simulink model "SF015A_WhlImbRejctn"  (R2013b)
settings: Solver=FixedStepDiscrete  SolverMode=SingleTasking  StartTime=0.0  StopTime=1  FixedStep=0.002  RelTol=1e-3
undefined symbols (not defined in the file): ACTIVBANDMAX_ULS_U32, ADAPVFILMAX_ULS_F32, ADJOUTPMAX_ULS_F32, ARCHGLBPRM_180OVERPI_ULS_F32, ARCHGLBPRM_2MILLISEC_SEC_F32, ARCHGLBPRM_2PI_ULS_F32, ARCHGLBPRM_FLOATZEROTHD_ULS_F32, ARCHGLBPRM_PI_ULS_F32, ARCHGLBPRM_PIOVER180_ULS_F32, ARCHGLBPRM_PIOVER2_ULS_F32, CALMINSPERCOUNT_ULS_F32, Cntr, DURATIONDISABLE_CNT_U16, FILTWHLSPDMAX_MOTRADPERSEC_F32, FRQMIN_ULS_F32, MICROSECTOMILLISEC_ULS_F32, MINSTOMILLISEC_ULS_F32, NINETY_ULS_F32, NODEBSTEP_CNT_U16, NROFDLY_CNT_U08, NtcSts1, NvmGetErrSts1, ONEHALF_ULS_F32, ONEHUNDRED_ULS_F32, ONEOVRTHREE_ULS_F32, ONEOVRTWENTY_ULS_F32, ONETHOUSAND_ULS_F32, PEAKMAX_ULS_F32, PEAKMIN_ULS_F32, PHAADJMAX_ULS_F32, PITIMESSAMPLETIME_ULS_F32, SigQlfr1, STOREDMINSPERCOUNT_ULS_F32, Sts, SysSt1, TWO_ULS_F32, TWOOVRTHREE_ULS_F32, UGRFILMAX_ULS_F32, WhlImbRejctnAdpvFac, WhlImbRejctnAutScaEna, WhlImbRejctnAutScaTar, WhlImbRejctnCurrMgnSlewPerLoop, WhlImbRejctnDcTrendFltRcvryDly, WhlImbRejctnDcTrendFltRcvryNegStep, WhlImbRejctnDcTrendFltRcvryPosStep, WhlImbRejctnDcTrendFltRcvryThd, WhlImbRejctnDcTrendTh2Tq, WhlImbRejctnDcTrendThTq, WhlImbRejctnDcTrendTi2Sec, WhlImbRejctnDcTrendTiSec, WhlImbRejctnEnaSlewPerLoop, WhlImbRejctnFctEna, WhlImbRejctnFltNtc, WhlImbRejctnFrqDiagcAmpThd, WhlImbRejctnFrqDiagcEna, WhlImbRejctnFrqDiagcFltRcvryDly, WhlImbRejctnFrqDiagcFltRcvryNegStep, WhlImbRejctnFrqDiagcFltRcvryPosStep, WhlImbRejctnFrqDiagcFltRcvryThd, WhlImbRejctnFrqDiagcThd ... (+30)
libraries: FixdToFloat x32, simulink x26, NxtrLim x25, Fil x20, NxtrAbslt x9, NxtrMath x7, NxtrMax x6, NxtrMin x4, NxtrNvM x2, FloatToFixd x2, LnrIntrpn x2, NxtrSign x1
(part 2 of 14)

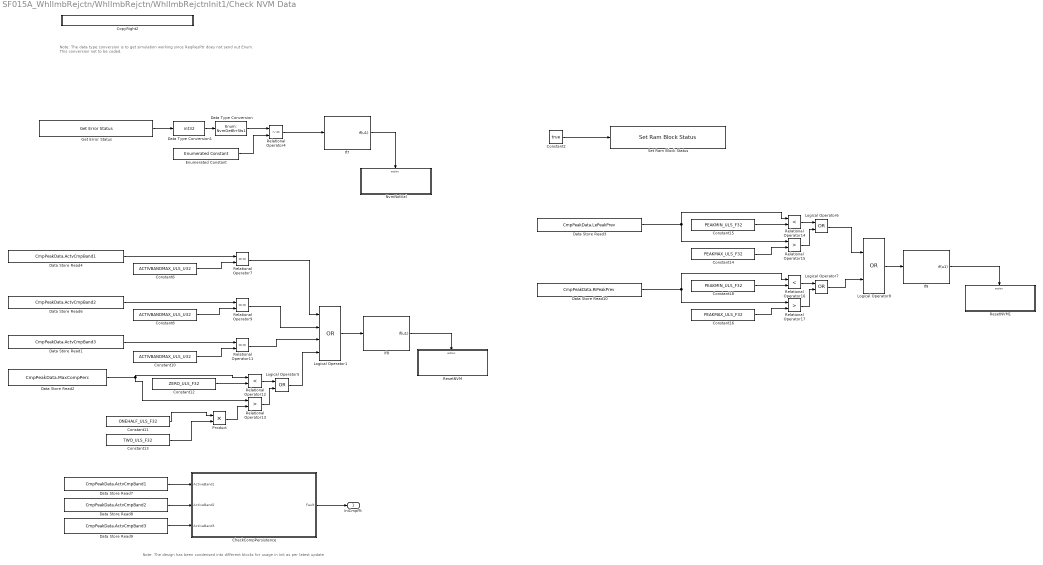
== system SF015A_WhlImbRejctn/WhlImbRejctn/WhlImbRejctnInit1/Check NVM Data ==
  note: Note: The data type conversion is to get simulation working since ReqResPtr does not send out Enum. This
      | conversion not to be coded.
  note: Note: The design has been condensed into different blocks for usage in Init as per latest update
  CheckCompPersistence : Subsystem
  Constant10 : Constant  RequirementInfo={} %GIDa_dac22d33_84e0_4d43_9baa_6580695156ec  Value=ACTIVBANDMAX_ULS_U32
  Constant11 : Constant  RequirementInfo={} %GIDa_b70b5de3_e4e7_4656_8a10_81d881ba1c41  Value=ONEHALF_ULS_F32
  Constant12 : Constant  RequirementInfo={} %GIDa_d9980660_ddd4_4231_a48f_0f3c433b1d8f  Value=ZERO_ULS_F32
  Constant13 : Constant  RequirementInfo={} %GIDa_8a202516_8579_4314_b780_b551ef6a9ea7  Value=TWO_ULS_F32
  Constant14 : Constant  RequirementInfo={} %GIDa_73aa9993_742b_457a_81a0_f953eb76670e  Value=PEAKMAX_ULS_F32
  Constant15 : Constant  RequirementInfo={} %GIDa_1412b3b4_8a5a_4483_b46c_39b8aea63137  Value=PEAKMIN_ULS_F32
  Constant16 : Constant  RequirementInfo={} %GIDa_fb2105b3_9180_4cca_ab02_2c62039e61f3  Value=PEAKMAX_ULS_F32
  Constant18 : Constant  RequirementInfo={} %GIDa_e66c83e2_3c4a_4c53_aaa1_18a5c79d3e74  Value=PEAKMIN_ULS_F32
  Constant2 : Constant  Value=true  OutDataTypeStr=boolean
      settings: AttributesFormatString=%<OutDataTypeStr>
  Constant6 : Constant  RequirementInfo={} %GIDa_8360f5ba_58c9_48ae_bbc1_d6eb240405df  Value=ACTIVBANDMAX_ULS_U32
  Constant8 : Constant  RequirementInfo={} %GIDa_5c7deeb0_1ebc_45b4_93cb_ec8df33bc324  Value=ACTIVBANDMAX_ULS_U32
  CopyRight2 : Subsystem  Description=|  mask(Copyright Information){none=on}
      | Copyright info block.                                               
      |                                                                     
      | Place copyright information at the top of every subsystem in design.
      mask prompts: none "No parameters"
      mask help: Place copyright information at the top of every subsystem in design.
      mask Display:
      | NxtrConf = 'Nexteer Confidential';
      | 
      | sys = bdroot; %handle for the current model ("system")
      | first = get_param(sys,'Created');
      | first = first(end-3:end);  %year is last four digits
      | 
      | last = get_param(sys,'LastModifiedDate');
      | if isempty(last)
      |     last = datestr(now,'yyyy');
      | else
      |     last = last(end-3:end);
      | end
      | 
      | if strcmp(first,last)
      |     fprintf('%s -- Copyright %s Nexteer',NxtrConf,first)
      | else
      |     fprintf('%s -- %s%s- %s Nexteer',NxtrConf,char(169),first,last)
      | end
  Data Store Read1 : DataStoreRead  RequirementInfo={} %GIDa_9fdfabdd_f7fe_4007_8b29_7d33a37c1ea7  DataStoreName=CmpPeakData  DataStoreElements=CmpPeakData.ActvCmpBand3
  Data Store Read10 : DataStoreRead  RequirementInfo={} %GIDa_8b90afc5_6e2e_402d_8a16_4fba91ced75f  DataStoreName=CmpPeakData  DataStoreElements=CmpPeakData.RiPeakPrev
  Data Store Read2 : DataStoreRead  RequirementInfo={} %GIDa_c9bc2b23_4b2d_4415_bc50_be739cb942b2  DataStoreName=CmpPeakData  DataStoreElements=CmpPeakData.MaxCompPerc
  Data Store Read3 : DataStoreRead  RequirementInfo={} %GIDa_b09638af_4375_4cc5_b3f9_eff43fa8b240  DataStoreName=CmpPeakData  DataStoreElements=CmpPeakData.LePeakPrev
  Data Store Read4 : DataStoreRead  RequirementInfo={} %GIDa_a896886f_cd25_4b88_9045_5429e28523e8  DataStoreName=CmpPeakData  DataStoreElements=CmpPeakData.ActvCmpBand1
  Data Store Read6 : DataStoreRead  RequirementInfo={} %GIDa_0bac01f8_9053_4f69_a3f3_2d14815d55fa  DataStoreName=CmpPeakData  DataStoreElements=CmpPeakData.ActvCmpBand2
  Data Store Read7 : DataStoreRead  Priority=3  DataStoreName=CmpPeakData  DataStoreElements=CmpPeakData.ActvCmpBand1
      settings: AttributesFormatString=Priority=%<Priority>
  Data Store Read8 : DataStoreRead  Priority=3  DataStoreName=CmpPeakData  DataStoreElements=CmpPeakData.ActvCmpBand2
      settings: AttributesFormatString=Priority=%<Priority>
  Data Store Read9 : DataStoreRead  Priority=3  DataStoreName=CmpPeakData  DataStoreElements=CmpPeakData.ActvCmpBand3
      settings: AttributesFormatString=Priority=%<Priority>
  Data Type Conversion : DataTypeConversion  RequirementInfo={} %GIDa_40af021a_ef54_4ec7_b6de_237be91b60fa  OutDataTypeStr=Enum: NvmGetErrSts1
  Data Type Conversion1 : DataTypeConversion  RequirementInfo={} %GIDa_97cfbfab_5bcd_4235_a187_9f25ba5a5ff5  OutDataTypeStr=int32
  Enumerated Constant : simulink/Sources/Enumerated Constant  RequirementInfo={} %GIDa_d56addf7_f0d4_4bf6_af4c_9a6eaaf5d064  OutDataTypeStr=Enum: NvmGetErrSts1  Value=NvmGetErrSts1.REQUEST_OK  SampleTime=inf
  Get Error Status : NxtrNvM/Get Error Status  RequirementInfo={} %GIDa_553b790d_fe60_40ec_8b91_d9fbb8c02471  FuncName=Get Error Status  NvMBlockName=CmpPeakData  VoidFuncRtn=on  ReqResPtr_DSN=NvMGES_ReqResPtr1  Return_DSN=NvMGES_Return
      settings: AttributesFormatString=%<FuncName>
  If7 : If  RequirementInfo={} %GIDa_907c88cf_d2cc_420d_8539_4883f54d5bfb  Priority=0  IfExpression=u1  ShowElse=off
  If8 : If  RequirementInfo={} %GIDa_f83260c7_70fe_47e6_bcfd_8d40190318cc  Priority=0  IfExpression=u1  ShowElse=off
  If9 : If  RequirementInfo={} %GIDa_2d76ece9_77c8_4d3b_9932_2561659afd1c  Priority=0  IfExpression=u1  ShowElse=off
  Logical Operator1 : Logic  RequirementInfo={} %GIDa_6b27fa6d_5a8c_4b6e_9ec1_9ce35c4a7e3a  Operator=OR  Inputs=4  AllPortsSameDT=off  OutDataTypeStr=boolean
  Logical Operator5 : Logic  RequirementInfo={} %GIDa_ff21cde4_e337_434b_869a_bfcb48407868  Operator=OR  AllPortsSameDT=off  OutDataTypeStr=boolean
  Logical Operator6 : Logic  RequirementInfo={} %GIDa_22490e7d_9c19_4dde_99cc_08f0ef37cc37  Operator=OR  AllPortsSameDT=off  OutDataTypeStr=boolean
  Logical Operator7 : Logic  RequirementInfo={} %GIDa_0952c7bd_6ac0_4128_a8d2_c4d9c59f71ec  Operator=OR  AllPortsSameDT=off  OutDataTypeStr=boolean
  Logical Operator8 : Logic  RequirementInfo={} %GIDa_f87f89e5_1919_41e6_b4c5_1617d795e711  Operator=OR  AllPortsSameDT=off  OutDataTypeStr=boolean
  NvmNotVal : Subsystem  RequirementInfo={} %GIDa_f6393af9_0f72_404f_ae39_57d92493339f  TreatAsAtomicUnit=on
  Product : Product
  Relational Operator11 : RelationalOperator  RequirementInfo={} %GIDa_9bbcc360_5740_4f1b_a35a_ba783374856a  Operator===  OutDataTypeStr=boolean
  Relational Operator12 : RelationalOperator  RequirementInfo={} %GIDa_a76e833d_5218_4e43_8d52_6f49a79e2f35  Operator=<  OutDataTypeStr=boolean
  Relational Operator13 : RelationalOperator  RequirementInfo={} %GIDa_4a8bae17_bbe3_48ac_9e0a_4fe9b537a9c6  Operator=>  OutDataTypeStr=boolean
  Relational Operator14 : RelationalOperator  RequirementInfo={} %GIDa_654c4bba_0100_4331_8452_58d1590c8b97  Operator=<  OutDataTypeStr=boolean
  Relational Operator15 : RelationalOperator  RequirementInfo={} %GIDa_e495d182_ff98_497d_82f4_fbf92eddef9e  Operator=>  OutDataTypeStr=boolean
  Relational Operator16 : RelationalOperator  RequirementInfo={} %GIDa_956274a6_c5b5_492b_bac4_f5c4aafd6507  Operator=<  OutDataTypeStr=boolean
  Relational Operator17 : RelationalOperator  RequirementInfo={} %GIDa_3a72db96_6452_4e24_94d0_249eb710d610  Operator=>  OutDataTypeStr=boolean
  Relational Operator4 : RelationalOperator  RequirementInfo={} %GIDa_240ffe86_9b38_40e3_a7e4_d3f8c5427260  Operator=~=  OutDataTypeStr=boolean
  Relational Operator7 : RelationalOperator  RequirementInfo={} %GIDa_ed9b8f8a_c888_45f6_bfd8_2fd8844e647e  Operator===  OutDataTypeStr=boolean
  Relational Operator9 : RelationalOperator  RequirementInfo={} %GIDa_5b0fe435_eb00_4504_b67e_fcbdb6466ad9  Operator===  OutDataTypeStr=boolean
  ResetNVM : Subsystem  RequirementInfo={} %GIDa_841a7b4b_65c9_4d3a_ad5a_ef4b7fb654a5  TreatAsAtomicUnit=on
  ResetNVM1 : Subsystem  RequirementInfo={} %GIDa_21072be2_221d_447f_a6c4_95766f8093de  TreatAsAtomicUnit=on
  Set Ram Block Status : NxtrNvM/Set Ram Block Status  FuncName=Set Ram Block Status  NvMBlockName=CmpPeakData  VoidFuncRtn=on  BlockChanged_DSN=NvMSRBS_BlockChanged1  Return_DSN=NvMSRBS_Return
  IniCmpFlt : Outport
  wires:
  Data Type Conversion/1 -> Relational Operator4/1
  Enumerated Constant/1 -> Relational Operator4/2
  Data Type Conversion1/1 -> Data Type Conversion/1
  Get Error Status/1 -> Data Type Conversion1/1
  Constant6/1 -> Relational Operator7/2
  Relational Operator7/1 -> Logical Operator1/1
  Constant8/1 -> Relational Operator9/2
  Constant10/1 -> Relational Operator11/2
  Logical Operator1/1 -> If8/1
  Data Store Read2/1 -> Relational Operator12/1, Relational Operator13/1
  Constant11/1 -> Product/1
  Constant12/1 -> Relational Operator12/2
  Relational Operator12/1 -> Logical Operator5/1
  Relational Operator13/1 -> Logical Operator5/2
  Logical Operator5/1 -> Logical Operator1/4
  Product/1 -> Relational Operator13/2
  Constant13/1 -> Product/2
  Data Store Read3/1 -> Relational Operator15/1, Relational Operator14/1
  Constant14/1 -> Relational Operator15/2
  Constant15/1 -> Relational Operator14/2
  Relational Operator14/1 -> Logical Operator6/1
  Relational Operator15/1 -> Logical Operator6/2
  Logical Operator6/1 -> Logical Operator8/1
  Data Store Read10/1 -> Relational Operator16/1, Relational Operator17/1
  Constant16/1 -> Relational Operator17/2
  Constant18/1 -> Relational Operator16/2
  Relational Operator16/1 -> Logical Operator7/1
  Relational Operator17/1 -> Logical Operator7/2
  Logical Operator7/1 -> Logical Operator8/2
  Logical Operator8/1 -> If9/1
  Relational Operator9/1 -> Logical Operator1/2
  Relational Operator11/1 -> Logical Operator1/3
  If7/1 -> NvmNotVal/Action
  If8/1 -> ResetNVM/Action
  If9/1 -> ResetNVM1/Action
  Data Store Read7/1 -> CheckCompPersistence/1(ActiveBand1)
  Data Store Read8/1 -> CheckCompPersistence/2(ActiveBand2)
  Data Store Read9/1 -> CheckCompPersistence/3(ActiveBand3)
  CheckCompPersistence/1(Fault) -> IniCmpFlt/1
  Data Store Read4/1 -> Relational Operator7/1
  Data Store Read6/1 -> Relational Operator9/1
  Data Store Read1/1 -> Relational Operator11/1
  Constant2/1 -> Set Ram Block Status/1
  Relational Operator4/1 -> If7/1

== system SF015A_WhlImbRejctn/WhlImbRejctn/WhlImbRejctnInit1/CopyRight2 ==

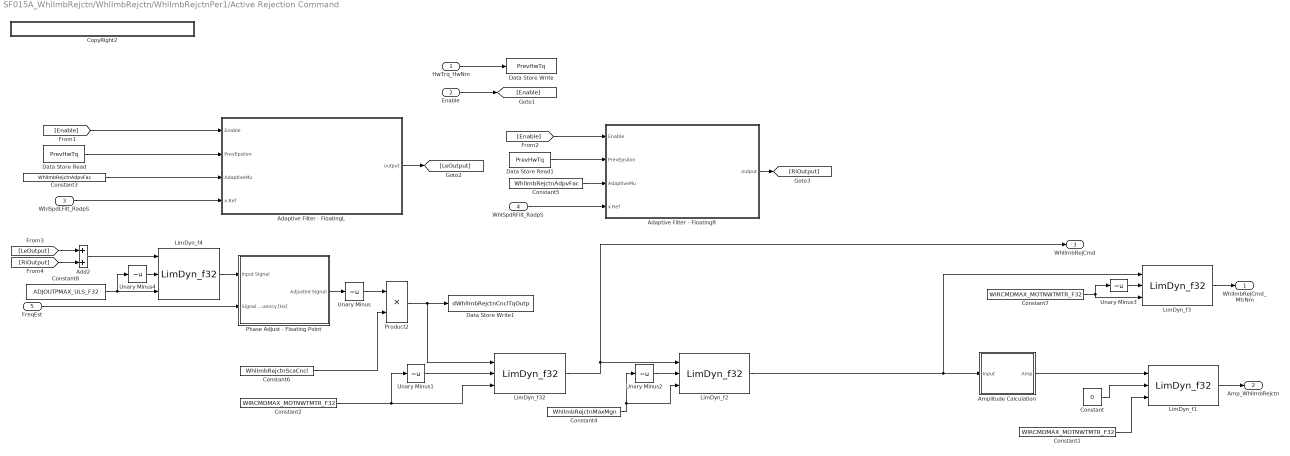
== system SF015A_WhlImbRejctn/WhlImbRejctn/WhlImbRejctnPer1/Active Rejection Command  ==
  HwTrq_HwNm : Inport
  Enable : Inport  Port=2
  WhlSpdLFilt_RadpS : Inport  Port=3
  WhlSpdRFilt_RadpS : Inport  Port=4
  FreqEst : Inport  Port=5
  Adaptive Filter - FloatingL : Subsystem
  Adaptive Filter - FloatingR : Subsystem
  Add2 : Sum
  Amplitude Calculation : Subsystem
  Constant : Constant  Value=0  OutDataTypeStr=single
  Constant1 : Constant  Value=WIRCMDMAX_MOTNWTMTR_F32
  Constant2 : Constant  Value=WIRCMDMAX_MOTNWTMTR_F32
  Constant3 : Constant  Value=WhlImbRejctnAdpvFac
  Constant4 : Constant  Value=WhlImbRejctnMaxMgn
  Constant5 : Constant  Value=WhlImbRejctnAdpvFac
  Constant6 : Constant  Value=WhlImbRejctnScaCncl
  Constant7 : Constant  Value=WIRCMDMAX_MOTNWTMTR_F32
  Constant8 : Constant  Value=ADJOUTPMAX_ULS_F32
  CopyRight2 : Subsystem  Description=|  mask(Copyright Information){none=on}
      | Copyright info block.                                               
      |                                                                     
      | Place copyright information at the top of every subsystem in design.
      mask prompts: none "No parameters"
      mask help: Place copyright information at the top of every subsystem in design.
      mask Display:
      | NxtrConf = 'Nexteer Confidential';
      | 
      | sys = bdroot; %handle for the current model ("system")
      | first = get_param(sys,'Created');
      | first = first(end-3:end);  %year is last four digits
      | 
      | last = get_param(sys,'LastModifiedDate');
      | if isempty(last)
      |     last = datestr(now,'yyyy');
      | else
      |     last = last(end-3:end);
      | end
      | 
      | if strcmp(first,last)
      |     fprintf('%s -- Copyright %s Nexteer',NxtrConf,first)
      | else
      |     fprintf('%s -- %s%s- %s Nexteer',NxtrConf,char(169),first,last)
      | end
  Data Store Read : DataStoreRead  Priority=1  DataStoreName=PrevHwTq
      settings: AttributesFormatString=%<Priority>
  Data Store Read1 : DataStoreRead  Priority=1  DataStoreName=PrevHwTq
      settings: AttributesFormatString=%<Priority>
  Data Store Write : DataStoreWrite  Priority=2  DataStoreName=PrevHwTq
      settings: AttributesFormatString=%<Priority>
  Data Store Write1 : DataStoreWrite  DataStoreName=dWhlImbRejctnCnclTqOutp
  LimDyn_f{1..4,32} (5 alike) : NxtrLim/LimDyn_f32
  Phase Adjust - Floating Point : Subsystem
  Product2 : Product
  Unary Minus{,1..4} (5 alike) : UnaryMinus
  WhlImbRejCmd_MtrNm : Outport
  Amp_WhlImbRejctn : Outport  Port=2
  WhlImbRejCmd : Outport  Port=3
  wires:
  FreqEst/1 -> Phase Adjust - Floating Point/2(Signal Frequency [Hz])
  Constant2/1 -> LimDyn_f32/3, Unary Minus1/1
  Unary Minus1/1 -> LimDyn_f32/2
  Data Store Read/1 -> Adaptive Filter - FloatingL/2(PrevEpsilon)
  Constant3/1 -> Adaptive Filter - FloatingL/3(AdaptiveMu)
  WhlSpdLFilt_RadpS/1 -> Adaptive Filter - FloatingL/4(x Ref)
  Data Store Read1/1 -> Adaptive Filter - FloatingR/2(PrevEpsilon)
  Constant5/1 -> Adaptive Filter - FloatingR/3(AdaptiveMu)
  WhlSpdRFilt_RadpS/1 -> Adaptive Filter - FloatingR/4(x Ref)
  Add2/1 -> LimDyn_f4/1
  Constant6/1 -> Product2/2
  Unary Minus/1 -> Product2/1
  Enable/1 -> [Enable]
  [Enable] -> Adaptive Filter - FloatingL/1(Enable)
  [Enable] -> Adaptive Filter - FloatingR/1(Enable)
  Adaptive Filter - FloatingL/1(output) -> [LeOutput]
  [LeOutput] -> Add2/1
  [RiOutput] -> Add2/2
  Adaptive Filter - FloatingR/1(output) -> [RiOutput]
  Phase Adjust - Floating Point/1(Adjusted Signal) -> Unary Minus/1
  HwTrq_HwNm/1 -> Data Store Write/1
  Product2/1 -> LimDyn_f32/1, Data Store Write1/1
  LimDyn_f2/1 -> LimDyn_f3/1, Amplitude Calculation/1(Input)
  LimDyn_f1/1 -> Amp_WhlImbRejctn/1
  Amplitude Calculation/1(Amp) -> LimDyn_f1/1
  Constant/1 -> LimDyn_f1/2
  Constant1/1 -> LimDyn_f1/3
  LimDyn_f4/1 -> Phase Adjust - Floating Point/1(Input Signal)
  Unary Minus4/1 -> LimDyn_f4/2
  Constant8/1 -> LimDyn_f4/3, Unary Minus4/1
  Unary Minus2/1 -> LimDyn_f2/2
  Constant4/1 -> Unary Minus2/1, LimDyn_f2/3
  LimDyn_f32/1 -> WhlImbRejCmd/1, LimDyn_f2/1
  Constant7/1 -> LimDyn_f3/3, Unary Minus3/1
  Unary Minus3/1 -> LimDyn_f3/2
  LimDyn_f3/1 -> WhlImbRejCmd_MtrNm/1

== system SF015A_WhlImbRejctn/WhlImbRejctn/WhlImbRejctnPer1/CopyRight2 ==

== system SF015A_WhlImbRejctn/WhlImbRejctn/WhlImbRejctnPer1/Determine Enabled Amt ==
  FreqEstAvg_Hz1 : Inport
  WhlSpdLFilt : Inport  Port=2
  WhlSpdRFilt : Inport  Port=3
  VehSpd : Inport  Port=4
  VehspdValid : Inport  Port=5
  WhlImbRejctnCustEna : Inport  Port=6
  WhlImbRejctnDi : Inport  Port=7
  System_State : Inport  Port=8
  CurrMgnSlewRate : Inport  Port=9
  EnaSlewRate : Inport  Port=10
  Calculate Enable1 : Subsystem
  CopyRight2 : Subsystem  Description=|  mask(Copyright Information){none=on}
      | Copyright info block.                                               
      |                                                                     
      | Place copyright information at the top of every subsystem in design.
      mask prompts: none "No parameters"
      mask help: Place copyright information at the top of every subsystem in design.
      mask Display:
      | NxtrConf = 'Nexteer Confidential';
      | 
      | sys = bdroot; %handle for the current model ("system")
      | first = get_param(sys,'Created');
      | first = first(end-3:end);  %year is last four digits
      | 
      | last = get_param(sys,'LastModifiedDate');
      | if isempty(last)
      |     last = datestr(now,'yyyy');
      | else
      |     last = last(end-3:end);
      | end
      | 
      | if strcmp(first,last)
      |     fprintf('%s -- Copyright %s Nexteer',NxtrConf,first)
      | else
      |     fprintf('%s -- %s%s- %s Nexteer',NxtrConf,char(169),first,last)
      | end
  Data Store Read : DataStoreRead  DataStoreName=RampYes
  Data Store Read1 : DataStoreRead  DataStoreName=RampNo
  Data Store Write1 : DataStoreWrite  DataStoreName=dWhlImbRejctnScaRi
  Data Store Write4 : DataStoreWrite  DataStoreName=dWhlImbRejctnScaLe
  Enable Ramp : Subsystem
  ScaleL : Outport
  ScaleR : Outport  Port=2
  Enable : Outport  Port=3
  WhlImbRejctnActv : Outport  Port=4
  wires:
  FreqEstAvg_Hz1/1 -> Calculate Enable1/1(FreqEstAvg_Hz)
  WhlSpdLFilt/1 -> Calculate Enable1/2(WhlSpdLFilt)
  WhlSpdRFilt/1 -> Calculate Enable1/3(WhlSpdRFilt)
  Calculate Enable1/2(ScaleR) -> Data Store Write1/1, ScaleR/1
  VehSpd/1 -> Calculate Enable1/4(Vehicle_Speed)
  VehspdValid/1 -> Calculate Enable1/5(Vehicle_Speed_Valid)
  WhlImbRejctnCustEna/1 -> Calculate Enable1/6(WhlImbRejctnCustEna)
  WhlImbRejctnDi/1 -> Calculate Enable1/7(WhlImbRejctnDi)
  Calculate Enable1/4(Enable) -> Enable Ramp/1(Enable In)
  Enable Ramp/1(Ramped Enable) -> Enable/1
  Calculate Enable1/1(ScaleL) -> Data Store Write4/1, ScaleL/1
  System_State/1 -> Enable Ramp/4(SYSTEM_STATE)
  Data Store Read/1 -> Enable Ramp/2("RampY ")
  Data Store Read1/1 -> Enable Ramp/3(RampN)
  Calculate Enable1/3(WhlImbRejctnActv) -> WhlImbRejctnActv/1
  CurrMgnSlewRate/1 -> Calculate Enable1/8(CurrMgnSlewRate)
  EnaSlewRate/1 -> Calculate Enable1/9(EnaSlewRate)

== system SF015A_WhlImbRejctn/WhlImbRejctn/WhlImbRejctnPer1/WIR Diagnostics ==
  note: Logic for setting of NTC bit based on WheelFrequencyValid
      | signal has been removed.
  CancelTrqOutput : Inport
  FreqEstAvg : Inport  Port=2
  EnabledComp : Inport  Port=3
  FreqR : Inport  Port=4
  FreqL : Inport  Port=5
  QualStat : Inport  Port=6
  "SlowSpeedDiagc " : Inport  Port=7
  IniCmpFlt : Inport  Port=8
  Amplitude Calculation1 : Subsystem
  CopyRight2 : Subsystem  Description=|  mask(Copyright Information){none=on}
      | Copyright info block.                                               
      |                                                                     
      | Place copyright information at the top of every subsystem in design.
      mask prompts: none "No parameters"
      mask help: Place copyright information at the top of every subsystem in design.
      mask Display:
      | NxtrConf = 'Nexteer Confidential';
      | 
      | sys = bdroot; %handle for the current model ("system")
      | first = get_param(sys,'Created');
      | first = first(end-3:end);  %year is last four digits
      | 
      | last = get_param(sys,'LastModifiedDate');
      | if isempty(last)
      |     last = datestr(now,'yyyy');
      | else
      |     last = last(end-3:end);
      | end
      | 
      | if strcmp(first,last)
      |     fprintf('%s -- Copyright %s Nexteer',NxtrConf,first)
      | else
      |     fprintf('%s -- %s%s- %s Nexteer',NxtrConf,char(169),first,last)
      | end
  Data Store Write : DataStoreWrite  DataStoreName=RampYes
  Data Store Write1 : DataStoreWrite  DataStoreName=RampNo
  DcTrendDiag : Subsystem
  FrequencyDiag : Subsystem
  If : If  IfExpression=u1
  Logical Operator1 : Logic  Operator=OR  Inputs=4  AllPortsSameDT=off  OutDataTypeStr=boolean
  Logical Operator2 : Logic  Operator=OR  Inputs=3  AllPortsSameDT=off  OutDataTypeStr=boolean
  Logical Operator3 : Logic  Operator=OR  Inputs=3  AllPortsSameDT=off  OutDataTypeStr=boolean
  Logical Operator4 : Logic  Operator=NOT  AllPortsSameDT=off  OutDataTypeStr=boolean
  Logical Operator5 : Logic  Operator=OR  AllPortsSameDT=off  OutDataTypeStr=boolean
  Logical Operator6 : Logic  Operator=OR  Inputs=3  AllPortsSameDT=off  OutDataTypeStr=boolean
  MaxMagDiag : Subsystem
  Set NTC Block : Subsystem  TreatAsAtomicUnit=on
  Set NTC Block1 : Subsystem  TreatAsAtomicUnit=on
  WhlSpdCorrDiag : Subsystem
  CmdAmp : Outport
  MaxMag : Outport  Port=2
  DCTrend : Outport  Port=3
  FrqDiagc : Outport  Port=4
  WhlSpdCorrln : Outport  Port=5
  wires:
  CancelTrqOutput/1 -> Amplitude Calculation1/1(Input), FrequencyDiag/1(WIRCmd), DcTrendDiag/1(WIRCmd)
  EnabledComp/1 -> FrequencyDiag/3(Enable)
  FreqEstAvg/1 -> FrequencyDiag/2(FreqEst)
  FreqR/1 -> WhlSpdCorrDiag/1(WhlFreqR)
  FreqL/1 -> WhlSpdCorrDiag/2(WhlFreqL)
  Amplitude Calculation1/1(Amp) -> CmdAmp/1, MaxMagDiag/1(CmdAmp), FrequencyDiag/4(CmdAmp)
  Logical Operator2/1 -> Data Store Write/1
  "SlowSpeedDiagc "/1 -> Logical Operator5/2, Logical Operator2/1
  Logical Operator3/1 -> If/1
  If/1 -> Set NTC Block/Action
  Logical Operator1/1 -> Data Store Write1/1
  QualStat/1 -> Logical Operator4/1
  Logical Operator4/1 -> Logical Operator1/4
  IniCmpFlt/1 -> Logical Operator2/3, Logical Operator5/1
  Logical Operator5/1 -> Set NTC Block/5(MaxPersis), Logical Operator3/3
  MaxMagDiag/1(FltStat) -> Set NTC Block/1(MaxMag), MaxMag/1, Logical Operator2/2, Logical Operator3/1
  DcTrendDiag/1(FltStat) -> Set NTC Block/2(DC Trend), DCTrend/1, Logical Operator1/1, Logical Operator6/1
  FrequencyDiag/1(FltStat) -> Set NTC Block/3(FrqDiagc), FrqDiagc/1, Logical Operator1/2, Logical Operator6/2
  WhlSpdCorrDiag/1(FltStat) -> Set NTC Block/4(WhlSpdCorrln), WhlSpdCorrln/1, Logical Operator1/3, Logical Operator6/3
  If/2 -> Set NTC Block1/Action
  Logical Operator6/1 -> Logical Operator3/2

== system SF015A_WhlImbRejctn/WhlImbRejctn/WhlImbRejctnPer1/Whl Spd filter and Freq Estimation ==
  QualWhlFreqL_Hz : Inport
  ScaleL : Inport  Port=2
  QualWhlFreqR_Hz : Inport  Port=3
  ScaleR : Inport  Port=4
  Add : Sum
  Constant : Constant  Value=FILTWHLSPDMAX_MOTRADPERSEC_F32
  Constant1 : Constant  Value=ARCHGLBPRM_2PI_ULS_F32
  Constant2 : Constant  Value=ARCHGLBPRM_2PI_ULS_F32
  Constant3 : Constant  Value=FILTWHLSPDMAX_MOTRADPERSEC_F32
  Constant4 : Constant  Value=WhlImbRejctnUgrPoleMgn
  Constant5 : Constant  Value=WhlImbRejctnUgrPoleMgn
  CopyRight2 : Subsystem  Description=|  mask(Copyright Information){none=on}
      | Copyright info block.                                               
      |                                                                     
      | Place copyright information at the top of every subsystem in design.
      mask prompts: none "No parameters"
      mask help: Place copyright information at the top of every subsystem in design.
      mask Display:
      | NxtrConf = 'Nexteer Confidential';
      | 
      | sys = bdroot; %handle for the current model ("system")
      | first = get_param(sys,'Created');
      | first = first(end-3:end);  %year is last four digits
      | 
      | last = get_param(sys,'LastModifiedDate');
      | if isempty(last)
      |     last = datestr(now,'yyyy');
      | else
      |     last = last(end-3:end);
      | end
      | 
      | if strcmp(first,last)
      |     fprintf('%s -- Copyright %s Nexteer',NxtrConf,first)
      | else
      |     fprintf('%s -- %s%s- %s Nexteer',NxtrConf,char(169),first,last)
      | end
  Data Store Write : DataStoreWrite  DataStoreName=StordValRi
  Data Store Write3 : DataStoreWrite  DataStoreName=dWhlImbRejctnFildWhlSpdRi
  Data Store Write4 : DataStoreWrite  DataStoreName=dWhlImbRejctnFildWhlSpdLe
  Data Store Write6 : DataStoreWrite  DataStoreName=StordValLe
  FilLpUpdOutp : Fil/FilLpUpdOutp  StVar=WhlSpdLeLpFil
      settings: AttributesFormatString=StVar: %<StVar>
  FilLpUpdOutp1 : Fil/FilLpUpdOutp  StVar=WhlSpdRiLpFil
      settings: AttributesFormatString=StVar: %<StVar>
  Gain : Gain  Gain=ONEHALF_ULS_F32
  LimDyn_f1 : NxtrLim/LimDyn_f32
  LimDyn_f32 : NxtrLim/LimDyn_f32
  Product{,1..3} (4 alike) : Product
  Tapped Delay ImplementationLe : Subsystem  TreatAsAtomicUnit=on
  Tapped Delay ImplementationRi : Subsystem  TreatAsAtomicUnit=on
  UGR L : Subsystem
  UGR R : Subsystem
  Unary Minus : UnaryMinus
  Unary Minus1 : UnaryMinus
  FiltWhlLSpd : Outport
  FiltWhlSpdLScld : Outport  Port=2
  FreqEst_Hz : Outport  Port=3
  FiltWhlRSpd : Outport  Port=4
  FiltWhlSpdRScld : Outport  Port=5
  wires:
  UGR L/1(y Filt) -> Product/1, LimDyn_f32/1, Data Store Write4/1
  FilLpUpdOutp/1 -> Add/1, UGR L/2(FreqEst_Hz)
  QualWhlFreqL_Hz/1 -> FilLpUpdOutp/1, Product3/2
  Product/1 -> Tapped Delay ImplementationLe/1(Input)
  ScaleL/1 -> Product/2
  Constant1/1 -> Product3/1
  Product3/1 -> UGR L/1(y)
  UGR R/1(y Filt) -> Product1/1, Data Store Write3/1, LimDyn_f1/1
  FilLpUpdOutp1/1 -> UGR R/2(FreqEst_Hz), Add/2
  QualWhlFreqR_Hz/1 -> FilLpUpdOutp1/1, Product2/2
  Product1/1 -> Tapped Delay ImplementationRi/1(Input)
  Constant2/1 -> Product2/1
  Product2/1 -> UGR R/1(y)
  ScaleR/1 -> Product1/2
  Add/1 -> Gain/1
  Gain/1 -> FreqEst_Hz/1
  Tapped Delay ImplementationRi/1(Tapped Signal) -> FiltWhlSpdRScld/1, Data Store Write/1
  Tapped Delay ImplementationLe/1(Tapped Signal) -> FiltWhlSpdLScld/1, Data Store Write6/1
  LimDyn_f32/1 -> FiltWhlLSpd/1
  Constant/1 -> Unary Minus/1, LimDyn_f32/3
  Unary Minus/1 -> LimDyn_f32/2
  LimDyn_f1/1 -> FiltWhlRSpd/1
  Constant3/1 -> Unary Minus1/1, LimDyn_f1/3
  Unary Minus1/1 -> LimDyn_f1/2
  Constant4/1 -> UGR L/3(PoleMag)
  Constant5/1 -> UGR R/3(PoleMag)

== system SF015A_WhlImbRejctn/WhlImbRejctn/WhlImbRejctnPer2/CopyRight2 ==

== system SF015A_WhlImbRejctn/WhlImbRejctn/WhlImbRejctnPer2/Flt Recovery- DC Trend ==
  FltStatIn : Inport
  FltRecDly : Inport  Port=2
  Constant : Constant  Value=MINSTOMILLISEC_ULS_F32
  CopyRight2 : Subsystem  Description=|  mask(Copyright Information){none=on}
      | Copyright info block.                                               
      |                                                                     
      | Place copyright information at the top of every subsystem in design.
      mask prompts: none "No parameters"
      mask help: Place copyright information at the top of every subsystem in design.
      mask Display:
      | NxtrConf = 'Nexteer Confidential';
      | 
      | sys = bdroot; %handle for the current model ("system")
      | first = get_param(sys,'Created');
      | first = first(end-3:end);  %year is last four digits
      | 
      | last = get_param(sys,'LastModifiedDate');
      | if isempty(last)
      |     last = datestr(now,'yyyy');
      | else
      |     last = last(end-3:end);
      | end
      | 
      | if strcmp(first,last)
      |     fprintf('%s -- Copyright %s Nexteer',NxtrConf,first)
      | else
      |     fprintf('%s -- %s%s- %s Nexteer',NxtrConf,char(169),first,last)
      | end
  Data Store Read : DataStoreRead  Priority=1  DataStoreName=DcTrendFltRcvry
      settings: AttributesFormatString=Priority:%<Priority>
  Data Store Write1 : DataStoreWrite  Priority=2  DataStoreName=DcTrendFltRcvry
      settings: AttributesFormatString=Priority:%<Priority>
  Data Store Write2 : DataStoreWrite  Priority=2  DataStoreName=DcTrendFltRst
      settings: AttributesFormatString=Priority:%<Priority>
  Divide : Product  Inputs=**
  ElapsedTime1 : Subsystem  TreatAsAtomicUnit=on
  FaultReset_Rcvry_False : Subsystem  TreatAsAtomicUnit=on
  FaultReset_Rcvry_True : Subsystem  TreatAsAtomicUnit=on
  If : If  IfExpression=u1
  Merge : Merge
  Relational Operator4 : RelationalOperator  OutDataTypeStr=boolean
  Update Fault Status : Subsystem  TreatAsAtomicUnit=on
  wires:
  ElapsedTime1/1(ElapsedTime) -> Relational Operator4/1
  FltStatIn/1 -> ElapsedTime1/1(FltStsTrue)
  FltRecDly/1 -> Divide/1
  Data Store Read/1 -> Update Fault Status/1(Structvar)
  Update Fault Status/1(Structvar_out) -> Data Store Write1/1
  Divide/1 -> Relational Operator4/2
  Constant/1 -> Divide/2
  Relational Operator4/1 -> If/1, Update Fault Status/2(Status)
  If/1 -> FaultReset_Rcvry_True/Action
  If/2 -> FaultReset_Rcvry_False/Action
  FaultReset_Rcvry_True/1(Out1) -> Merge/1
  FaultReset_Rcvry_False/1(Out1) -> Merge/2
  Merge/1 -> Data Store Write2/1

== system SF015A_WhlImbRejctn/WhlImbRejctn/WhlImbRejctnPer2/Flt Recovery- Freq Diag ==
  FltStatIn : Inport
  FltRecDly : Inport  Port=2
  Constant : Constant  Value=MINSTOMILLISEC_ULS_F32
  CopyRight2 : Subsystem  Description=|  mask(Copyright Information){none=on}
      | Copyright info block.                                               
      |                                                                     
      | Place copyright information at the top of every subsystem in design.
      mask prompts: none "No parameters"
      mask help: Place copyright information at the top of every subsystem in design.
      mask Display:
      | NxtrConf = 'Nexteer Confidential';
      | 
      | sys = bdroot; %handle for the current model ("system")
      | first = get_param(sys,'Created');
      | first = first(end-3:end);  %year is last four digits
      | 
      | last = get_param(sys,'LastModifiedDate');
      | if isempty(last)
      |     last = datestr(now,'yyyy');
      | else
      |     last = last(end-3:end);
      | end
      | 
      | if strcmp(first,last)
      |     fprintf('%s -- Copyright %s Nexteer',NxtrConf,first)
      | else
      |     fprintf('%s -- %s%s- %s Nexteer',NxtrConf,char(169),first,last)
      | end
  Data Store Read : DataStoreRead  Priority=1  DataStoreName=FrqDiagcFltRcvry
      settings: AttributesFormatString=Priority:%<Priority>
  Data Store Write1 : DataStoreWrite  Priority=2  DataStoreName=FrqDiagcFltRcvry
      settings: AttributesFormatString=Priority:%<Priority>
  Data Store Write2 : DataStoreWrite  Priority=2  DataStoreName=FrqDiagcFltRst
      settings: AttributesFormatString=Priority:%<Priority>
  Divide : Product  Inputs=**
  ElapsedTime1 : Subsystem  TreatAsAtomicUnit=on
  FaultReset_Rcvry_False : Subsystem  TreatAsAtomicUnit=on
  FaultReset_Rcvry_True : Subsystem  TreatAsAtomicUnit=on
  If : If  IfExpression=u1
  Merge : Merge
  Relational Operator4 : RelationalOperator  OutDataTypeStr=boolean
  Update Fault Status : Subsystem  TreatAsAtomicUnit=on
  wires:
  ElapsedTime1/1(ElapsedTime) -> Relational Operator4/1
  FltStatIn/1 -> ElapsedTime1/1(FltStsTrue)
  FltRecDly/1 -> Divide/1
  Data Store Read/1 -> Update Fault Status/1(Structvar)
  Update Fault Status/1(Structvar_out) -> Data Store Write1/1
  Divide/1 -> Relational Operator4/2
  Constant/1 -> Divide/2
  Relational Operator4/1 -> If/1, Update Fault Status/2(Status)
  If/1 -> FaultReset_Rcvry_True/Action
  If/2 -> FaultReset_Rcvry_False/Action
  FaultReset_Rcvry_True/1(Out1) -> Merge/1
  FaultReset_Rcvry_False/1(Out1) -> Merge/2
  Merge/1 -> Data Store Write2/1

== system SF015A_WhlImbRejctn/WhlImbRejctn/WhlImbRejctnPer2/Flt Recovery- Max Mag ==
  FltStatIn : Inport
  FltRecDly : Inport  Port=2
  Constant : Constant  Value=MINSTOMILLISEC_ULS_F32
  CopyRight2 : Subsystem  Description=|  mask(Copyright Information){none=on}
      | Copyright info block.                                               
      |                                                                     
      | Place copyright information at the top of every subsystem in design.
      mask prompts: none "No parameters"
      mask help: Place copyright information at the top of every subsystem in design.
      mask Display:
      | NxtrConf = 'Nexteer Confidential';
      | 
      | sys = bdroot; %handle for the current model ("system")
      | first = get_param(sys,'Created');
      | first = first(end-3:end);  %year is last four digits
      | 
      | last = get_param(sys,'LastModifiedDate');
      | if isempty(last)
      |     last = datestr(now,'yyyy');
      | else
      |     last = last(end-3:end);
      | end
      | 
      | if strcmp(first,last)
      |     fprintf('%s -- Copyright %s Nexteer',NxtrConf,first)
      | else
      |     fprintf('%s -- %s%s- %s Nexteer',NxtrConf,char(169),first,last)
      | end
  Data Store Read : DataStoreRead  Priority=1  DataStoreName=MaxMgnFltRcvry
      settings: AttributesFormatString=Priority:%<Priority>
  Data Store Write1 : DataStoreWrite  Priority=2  DataStoreName=MaxMgnFltRcvry
      settings: AttributesFormatString=Priority:%<Priority>
  Data Store Write2 : DataStoreWrite  Priority=2  DataStoreName=MaxMgnFltRst
      settings: AttributesFormatString=Priority:%<Priority>
  Divide : Product  Inputs=**
  ElapsedTime1 : Subsystem  TreatAsAtomicUnit=on
  FaultReset_Rcvry_False : Subsystem  TreatAsAtomicUnit=on
  FaultReset_Rcvry_True : Subsystem  TreatAsAtomicUnit=on
  If : If  IfExpression=u1
  Merge : Merge
  Relational Operator4 : RelationalOperator  OutDataTypeStr=boolean
  Update Fault Status : Subsystem  TreatAsAtomicUnit=on
  wires:
  ElapsedTime1/1(ElapsedTime) -> Relational Operator4/1
  FltStatIn/1 -> ElapsedTime1/1(FltStsTrue)
  FltRecDly/1 -> Divide/1
  Data Store Read/1 -> Update Fault Status/1(Structvar)
  Update Fault Status/1(Structvar_out) -> Data Store Write1/1
  Divide/1 -> Relational Operator4/2
  Constant/1 -> Divide/2
  If/1 -> FaultReset_Rcvry_True/Action
  If/2 -> FaultReset_Rcvry_False/Action
  FaultReset_Rcvry_True/1(Out1) -> Merge/1
  FaultReset_Rcvry_False/1(Out1) -> Merge/2
  Merge/1 -> Data Store Write2/1
  Relational Operator4/1 -> If/1, Update Fault Status/2(Status)

== system SF015A_WhlImbRejctn/WhlImbRejctn/WhlImbRejctnPer2/Flt Recovery- WhlSpdCorr Diag ==
  FltStatIn : Inport
  FltRecDly : Inport  Port=2
  Constant : Constant  Value=MINSTOMILLISEC_ULS_F32
  CopyRight2 : Subsystem  Description=|  mask(Copyright Information){none=on}
      | Copyright info block.                                               
      |                                                                     
      | Place copyright information at the top of every subsystem in design.
      mask prompts: none "No parameters"
      mask help: Place copyright information at the top of every subsystem in design.
      mask Display:
      | NxtrConf = 'Nexteer Confidential';
      | 
      | sys = bdroot; %handle for the current model ("system")
      | first = get_param(sys,'Created');
      | first = first(end-3:end);  %year is last four digits
      | 
      | last = get_param(sys,'LastModifiedDate');
      | if isempty(last)
      |     last = datestr(now,'yyyy');
      | else
      |     last = last(end-3:end);
      | end
      | 
      | if strcmp(first,last)
      |     fprintf('%s -- Copyright %s Nexteer',NxtrConf,first)
      | else
      |     fprintf('%s -- %s%s- %s Nexteer',NxtrConf,char(169),first,last)
      | end
  Data Store Read : DataStoreRead  Priority=1  DataStoreName=WhlSpdCorrlnFltRcvry
      settings: AttributesFormatString=Priority:%<Priority>
  Data Store Write1 : DataStoreWrite  Priority=2  DataStoreName=WhlSpdCorrlnFltRcvry
      settings: AttributesFormatString=Priority:%<Priority>
  Data Store Write2 : DataStoreWrite  Priority=2  DataStoreName=WhlSpdCorrFltRst
      settings: AttributesFormatString=Priority:%<Priority>
  Divide : Product  Inputs=**
  ElapsedTime1 : Subsystem  TreatAsAtomicUnit=on
  FaultReset_Rcvry_False : Subsystem  TreatAsAtomicUnit=on
  FaultReset_Rcvry_True : Subsystem  TreatAsAtomicUnit=on
  If : If  IfExpression=u1
  Merge : Merge
  Relational Operator4 : RelationalOperator  OutDataTypeStr=boolean
  Update Fault Status : Subsystem  TreatAsAtomicUnit=on
  wires:
  ElapsedTime1/1(ElapsedTime) -> Relational Operator4/1
  FltStatIn/1 -> ElapsedTime1/1(FltStsTrue)
  FltRecDly/1 -> Divide/1
  Data Store Read/1 -> Update Fault Status/1(Structvar)
  Update Fault Status/1(Structvar_out) -> Data Store Write1/1
  Divide/1 -> Relational Operator4/2
  Constant/1 -> Divide/2
  Relational Operator4/1 -> If/1, Update Fault Status/2(Status)
  If/1 -> FaultReset_Rcvry_True/Action
  If/2 -> FaultReset_Rcvry_False/Action
  FaultReset_Rcvry_True/1(Out1) -> Merge/1
  FaultReset_Rcvry_False/1(Out1) -> Merge/2
  Merge/1 -> Data Store Write2/1

== system SF015A_WhlImbRejctn/WhlImbRejctn/WhlImbRejctnPer2/WIR Low Speed Diagnostics ==
  CmdAmp : Inport
  CopyRight2 : Subsystem  Description=|  mask(Copyright Information){none=on}
      | Copyright info block.                                               
      |                                                                     
      | Place copyright information at the top of every subsystem in design.
      mask prompts: none "No parameters"
      mask help: Place copyright information at the top of every subsystem in design.
      mask Display:
      | NxtrConf = 'Nexteer Confidential';
      | 
      | sys = bdroot; %handle for the current model ("system")
      | first = get_param(sys,'Created');
      | first = first(end-3:end);  %year is last four digits
      | 
      | last = get_param(sys,'LastModifiedDate');
      | if isempty(last)
      |     last = datestr(now,'yyyy');
      | else
      |     last = last(end-3:end);
      | end
      | 
      | if strcmp(first,last)
      |     fprintf('%s -- Copyright %s Nexteer',NxtrConf,first)
      | else
      |     fprintf('%s -- %s%s- %s Nexteer',NxtrConf,char(169),first,last)
      | end
  MaxPersisDiag : Subsystem
  WIRFltStatus_SlowSpeed : Outport
  wires:
  CmdAmp/1 -> MaxPersisDiag/1(CmdAmp)
  MaxPersisDiag/1(MaxPersistence_fault) -> WIRFltStatus_SlowSpeed/1

== system SF015A_WhlImbRejctn/WhlImbRejctn/WhlImbRejctnInit1/Check NVM Data/CheckCompPersistence ==
  ActiveBand1 : Inport
  ActiveBand2 : Inport  Port=2
  ActiveBand3 : Inport  Port=3
  Constant1 : Constant  Value=WhlImbRejctnMaxDurn
  Constant15 : Constant  Value=0  OutDataTypeStr=boolean
  Constant3 : Constant  Value=DURATIONDISABLE_CNT_U16
  CopyRight2 : Subsystem  Description=|  mask(Copyright Information){none=on}
      | Copyright info block.                                               
      |                                                                     
      | Place copyright information at the top of every subsystem in design.
      mask prompts: none "No parameters"
      mask help: Place copyright information at the top of every subsystem in design.
      mask Display:
      | NxtrConf = 'Nexteer Confidential';
      | 
      | sys = bdroot; %handle for the current model ("system")
      | first = get_param(sys,'Created');
      | first = first(end-3:end);  %year is last four digits
      | 
      | last = get_param(sys,'LastModifiedDate');
      | if isempty(last)
      |     last = datestr(now,'yyyy');
      | else
      |     last = last(end-3:end);
      | end
      | 
      | if strcmp(first,last)
      |     fprintf('%s -- Copyright %s Nexteer',NxtrConf,first)
      | else
      |     fprintf('%s -- %s%s- %s Nexteer',NxtrConf,char(169),first,last)
      | end
  Data Type Conversion1 : DataTypeConversion  OutDataTypeStr=boolean
  If1 : If  IfExpression=u1
  Merge5 : Merge
  NoFault : Subsystem  RequirementInfo={} %GIDa_ba94ca7d_ee6a_41fe_9637_ca38a72bc55f  TreatAsAtomicUnit=on
  Relational Operator1 : RelationalOperator  Operator=<=  OutDataTypeStr=boolean
  Subsystem : Subsystem
  Fault : Outport
  wires:
  Constant1/1 -> Relational Operator1/1
  Relational Operator1/1 -> If1/1
  Constant3/1 -> Relational Operator1/2
  If1/1 -> Subsystem/Action
  ActiveBand1/1 -> Subsystem/1(Band)
  ActiveBand2/1 -> Subsystem/2(Band2)
  ActiveBand3/1 -> Subsystem/3(Band3)
  Merge5/1 -> Fault/1
  Subsystem/1(Fault) -> Merge5/1
  Constant15/1 -> Data Type Conversion1/1
  NoFault/1(Output) -> Merge5/2
  If1/2 -> NoFault/Action
  Data Type Conversion1/1 -> NoFault/1(Input)

== system SF015A_WhlImbRejctn/WhlImbRejctn/WhlImbRejctnInit1/Check NVM Data/CopyRight2 ==

== system SF015A_WhlImbRejctn/WhlImbRejctn/WhlImbRejctnInit1/Check NVM Data/NvmNotVal ==
  Action Port : ActionPort  ActionType=then
  Constant : Constant  Value=ZERO_ULS_F32
  CopyRight2 : Subsystem  Description=|  mask(Copyright Information){none=on}
      | Copyright info block.                                               
      |                                                                     
      | Place copyright information at the top of every subsystem in design.
      mask prompts: none "No parameters"
      mask help: Place copyright information at the top of every subsystem in design.
      mask Display:
      | NxtrConf = 'Nexteer Confidential';
      | 
      | sys = bdroot; %handle for the current model ("system")
      | first = get_param(sys,'Created');
      | if(isempty(first))
      |     first = datestr(now,'yyyy');
      | else
      |     first = first(end-3:end);  %year is last four digits
      | end
      | 
      | last = get_param(sys,'LastModifiedDate');
      | if isempty(last)
      |     last = datestr(now,'yyyy');
      | else
      |     last = last(end-3:end);
      | end
      | 
      | if strcmp(first,last)
      |     fprintf('%s -- Copyright %s Nexteer',NxtrConf,first)
      | else
      |     fprintf('%s -- %s%s- %s Nexteer',NxtrConf,char(169),first,last)
      | end
  Data Store Write10 : DataStoreWrite  DataStoreName=CmpPeakData  DataStoreElements=CmpPeakData.RiPeakPrev
  Data Store Write3 : DataStoreWrite  DataStoreName=CmpPeakData  DataStoreElements=CmpPeakData.ActvCmpBand1
  Data Store Write6 : DataStoreWrite  DataStoreName=CmpPeakData  DataStoreElements=CmpPeakData.ActvCmpBand2
  Data Store Write7 : DataStoreWrite  DataStoreName=CmpPeakData  DataStoreElements=CmpPeakData.ActvCmpBand3
  Data Store Write8 : DataStoreWrite  DataStoreName=CmpPeakData  DataStoreElements=CmpPeakData.MaxCompPerc
  Data Store Write9 : DataStoreWrite  DataStoreName=CmpPeakData  DataStoreElements=CmpPeakData.LePeakPrev
  Data Type Conversion : DataTypeConversion  OutDataTypeStr=uint32
  Data Type Conversion1 : DataTypeConversion  OutDataTypeStr=uint32
  Data Type Conversion2 : DataTypeConversion  OutDataTypeStr=uint32
  wires:
  Constant/1 -> Data Type Conversion1/1, Data Store Write10/1, Data Store Write9/1, Data Store Write8/1, Data Type Conversion2/1, Data Type Conversion/1
  Data Type Conversion/1 -> Data Store Write3/1
  Data Type Conversion1/1 -> Data Store Write6/1
  Data Type Conversion2/1 -> Data Store Write7/1

== system SF015A_WhlImbRejctn/WhlImbRejctn/WhlImbRejctnInit1/Check NVM Data/ResetNVM ==
  Action Port : ActionPort  ActionType=then
  Constant : Constant  Value=ZERO_ULS_F32
  CopyRight2 : Subsystem  Description=|  mask(Copyright Information){none=on}
      | Copyright info block.                                               
      |                                                                     
      | Place copyright information at the top of every subsystem in design.
      mask prompts: none "No parameters"
      mask help: Place copyright information at the top of every subsystem in design.
      mask Display:
      | NxtrConf = 'Nexteer Confidential';
      | 
      | sys = bdroot; %handle for the current model ("system")
      | first = get_param(sys,'Created');
      | if(isempty(first))
      |     first = datestr(now,'yyyy');
      | else
      |     first = first(end-3:end);  %year is last four digits
      | end
      | 
      | last = get_param(sys,'LastModifiedDate');
      | if isempty(last)
      |     last = datestr(now,'yyyy');
      | else
      |     last = last(end-3:end);
      | end
      | 
      | if strcmp(first,last)
      |     fprintf('%s -- Copyright %s Nexteer',NxtrConf,first)
      | else
      |     fprintf('%s -- %s%s- %s Nexteer',NxtrConf,char(169),first,last)
      | end
  Data Store Write : DataStoreWrite  DataStoreName=CmpPeakData  DataStoreElements=CmpPeakData.ActvCmpBand2
  Data Store Write2 : DataStoreWrite  DataStoreName=CmpPeakData  DataStoreElements=CmpPeakData.ActvCmpBand3
  Data Store Write3 : DataStoreWrite  DataStoreName=CmpPeakData  DataStoreElements=CmpPeakData.MaxCompPerc
  Data Store Write4 : DataStoreWrite  DataStoreName=CmpPeakData  DataStoreElements=CmpPeakData.ActvCmpBand1
  Data Type Conversion : DataTypeConversion  OutDataTypeStr=uint32
  Data Type Conversion1 : DataTypeConversion  OutDataTypeStr=uint32
  Data Type Conversion2 : DataTypeConversion  OutDataTypeStr=uint32
  wires:
  Constant/1 -> Data Store Write3/1, Data Type Conversion2/1, Data Type Conversion1/1, Data Type Conversion/1
  Data Type Conversion/1 -> Data Store Write4/1
  Data Type Conversion1/1 -> Data Store Write/1
  Data Type Conversion2/1 -> Data Store Write2/1

== system SF015A_WhlImbRejctn/WhlImbRejctn/WhlImbRejctnInit1/Check NVM Data/ResetNVM1 ==
  Action Port : ActionPort  ActionType=then
  Constant : Constant  Value=ZERO_ULS_F32
  CopyRight2 : Subsystem  Description=|  mask(Copyright Information){none=on}
      | Copyright info block.                                               
      |                                                                     
      | Place copyright information at the top of every subsystem in design.
      mask prompts: none "No parameters"
      mask help: Place copyright information at the top of every subsystem in design.
      mask Display:
      | NxtrConf = 'Nexteer Confidential';
      | 
      | sys = bdroot; %handle for the current model ("system")
      | first = get_param(sys,'Created');
      | if(isempty(first))
      |     first = datestr(now,'yyyy');
      | else
      |     first = first(end-3:end);  %year is last four digits
      | end
      | 
      | last = get_param(sys,'LastModifiedDate');
      | if isempty(last)
      |     last = datestr(now,'yyyy');
      | else
      |     last = last(end-3:end);
      | end
      | 
      | if strcmp(first,last)
      |     fprintf('%s -- Copyright %s Nexteer',NxtrConf,first)
      | else
      |     fprintf('%s -- %s%s- %s Nexteer',NxtrConf,char(169),first,last)
      | end
  Data Store Write4 : DataStoreWrite  DataStoreName=CmpPeakData  DataStoreElements=CmpPeakData.RiPeakPrev
  Data Store Write5 : DataStoreWrite  DataStoreName=CmpPeakData  DataStoreElements=CmpPeakData.LePeakPrev
  wires:
  Constant/1 -> Data Store Write5/1, Data Store Write4/1
